simulink model "CMU_BORG_AplysiaModularNeuromechanics"  (R2024a)
settings: Solver=ode23  StartTime=0.0  StopTime=tend  FixedStep=0.001  MaxStep=0.1  RelTol=0.00001  AbsTol=0.0001
values from neighbouring files (symbols this model uses):
  B20_0 = 0    [ParameterRecalculation.m]    (also in ReferenceGeometry_and_Initialization.m)
  B31B32_0 = 0    [GetSteadyState.m]    (also in ParameterRecalculation.m = 1; ReferenceGeometry_and_Initialization.m = 1; VaryingSeaweedStrength.m = 1)
  B38_0 = 0    [ParameterRecalculation.m]    (also in ReferenceGeometry_and_Initialization.m)
  B40B30_0 = 0    [ParameterRecalculation.m]    (also in ReferenceGeometry_and_Initialization.m)
  B40B30_offTime_0 = 0    [ParameterRecalculation.m]    (also in ReferenceGeometry_and_Initialization.m)
  B43B45_0 = 0    [ParameterRecalculation.m]    (also in ReferenceGeometry_and_Initialization.m)
  B4B5_0 = 0    [ParameterRecalculation.m]    (also in ReferenceGeometry_and_Initialization.m)
  B64_0 = 1    [GetSteadyState.m]    (also in ParameterRecalculation.m = 0; ReferenceGeometry_and_Initialization.m = 0; VaryingSeaweedStrength.m = 0)
  B6B9B3_0 = 1    [GetSteadyState.m]    (also in ParameterRecalculation.m = 0; ReferenceGeometry_and_Initialization.m = 0; VaryingSeaweedStrength.m = 0)
  B7_0 = 0    [ParameterRecalculation.m]    (also in ReferenceGeometry_and_Initialization.m)
  B8_0 = 0    [ParameterRecalculation.m]    (also in ReferenceGeometry_and_Initialization.m)
  C1_0 = 0    [ParameterRecalculation.m]    (also in ReferenceGeometry_and_Initialization.m)
  C2_0 = 0    [ParameterRecalculation.m]    (also in ReferenceGeometry_and_Initialization.m)
  C6_0 = 0    [ParameterRecalculation.m]    (also in ReferenceGeometry_and_Initialization.m)
  C_theta = C_xg/(2*pi)    [ParameterRecalculation.m]    (also in ReferenceGeometry_and_Initialization.m = 0.000813600069086)
  C_xd = C_xg    [ParameterRecalculation.m]    (also in ReferenceGeometry_and_Initialization.m = 0.005112)
  C_xg = (1/inv_C(kk))*time_scaler*force_scaler    [DampingParameterConvergence.m]    (also in ReferenceGeometry_and_Initialization.m = 0.005112)
  C_xv = C_xd    [ParameterRecalculation.m]    (also in ReferenceGeometry_and_Initialization.m = 0.005112)
  C_yg = C_xg    [ParameterRecalculation.m]    (also in ReferenceGeometry_and_Initialization.m = 0.005112)
  CBI2_0 = 0    [ParameterRecalculation.m]    (also in ReferenceGeometry_and_Initialization.m)
  CBI3_0 = 0    [GetSteadyState.m]    (also in ParameterRecalculation.m = 1; ReferenceGeometry_and_Initialization.m = 1; VaryingSeaweedStrength.m = 1)
  CBI3_refractory_0 = 0    [ParameterRecalculation.m]    (also in ReferenceGeometry_and_Initialization.m)
  CBI3_stimOFF_0 = 0    [ParameterRecalculation.m]    (also in ReferenceGeometry_and_Initialization.m)
  CBI3_stimON_0 = 0    [ParameterRecalculation.m]    (also in ReferenceGeometry_and_Initialization.m)
  CBI4_0 = 0    [ParameterRecalculation.m]    (also in ReferenceGeometry_and_Initialization.m)
  E1_params = [AE10,TE10,tau_E1,L0_E1,Lmax_E1]    [ParameterRecalculation.m]    (also in ReferenceGeometry_and_Initialization.m)
  E2_params = [AE20,TE20,tau_E2,L0_E2,Lmax_E2]    [ParameterRecalculation.m]    (also in ReferenceGeometry_and_Initialization.m)
  E6_params = [AE60,TE60,tau_E6,L0_E6,Lmax_E6]    [ParameterRecalculation.m]    (also in ReferenceGeometry_and_Initialization.m)
  FE1_max = force_scaler*0.2    [ParameterRecalculation.m]    (also in ReferenceGeometry_and_Initialization.m = 0.048)
  FE2_max = FE1_max    [ParameterRecalculation.m]    (also in ReferenceGeometry_and_Initialization.m = 0.048)
  FE6_max = FE1_max    [ParameterRecalculation.m]    (also in ReferenceGeometry_and_Initialization.m = 0.048)
  FHinge_max = force_scaler*0.292    [ParameterRecalculation.m]    (also in ReferenceGeometry_and_Initialization.m = 0.07008)
  FI1d_max = force_scaler*3.2    [ParameterRecalculation.m]    (also in ReferenceGeometry_and_Initialization.m = 0.768)
  FI1v_max = FI1d_max    [ParameterRecalculation.m]    (also in ReferenceGeometry_and_Initialization.m = 0.768)
  FI2_max = force_scaler*1    [ParameterRecalculation.m]    (also in ReferenceGeometry_and_Initialization.m = 0.24)
  FI3_ant_max = force_scaler*0.1    [ParameterRecalculation.m]    (also in ReferenceGeometry_and_Initialization.m = 0.024)
  FI3_max = force_scaler*3    [ParameterRecalculation.m]    (also in ReferenceGeometry_and_Initialization.m = 0.72)
  FI4_max = force_scaler*0.9    [ParameterRecalculation.m]    (also in ReferenceGeometry_and_Initialization.m = 0.216)
  fixation_type = 0    [GetSteadyState.m]    (also in ModelController.m; VaryingSeaweedStrength.m)
  grasperR = 1    [ReferenceGeometry_and_Initialization.m]
  H_lumen = mean([L_jaw,L_LG]) / R_ref    [ReferenceGeometry_and_Initialization.m]
  Hinge_params = [A_hinge0,T_hinge0,tau_hinge,L0_hinge,Lmax_hinge]    [ParameterRecalculation.m]    (also in ReferenceGeometry_and_Initialization.m)
  I1d_params = [AI1d0,TI1d0,tau_I1d,L0_I1d,Lmax_I1d]    [ParameterRecalculation.m]    (also in ReferenceGeometry_and_Initialization.m)
  I1v_params = [AI1v0,TI1v0,tau_I1v,L0_I1v,Lmax_I1v]    [ParameterRecalculation.m]    (also in ReferenceGeometry_and_Initialization.m)
  I2_params = [AI20,TI20,tau_I2_ingestive,tau_I2_egestive,L0_I2,Lmax_I2]    [ParameterRecalculation.m]    (also in ReferenceGeometry_and_Initialization.m)
  I3_params = [AI30,TI30,tau_I3]    [ParameterRecalculation.m]    (also in ReferenceGeometry_and_Initialization.m)
  I3ant_params = [AI3_ant0,TI3_ant0,tau_I3ant]    [ParameterRecalculation.m]    (also in ReferenceGeometry_and_Initialization.m)
  I4_params = [AI40,TI40,tau_I4]    [ParameterRecalculation.m]    (also in ReferenceGeometry_and_Initialization.m)
  K_const = force_scaler*0.5    [ParameterRecalculation.m]    (also in ReferenceGeometry_and_Initialization.m = 0.12)
  K_Eso = force_scaler*0.01    [ParameterRecalculation.m]    (also in ReferenceGeometry_and_Initialization.m = 0.0024)
  K_H = force_scaler*2    [ParameterRecalculation.m]    (also in ReferenceGeometry_and_Initialization.m = 0.48)
  L0_eso = abs(xd0)    [ReferenceGeometry_and_Initialization.m]
  L0_H = 0    [ReferenceGeometry_and_Initialization.m]
  L0_I1d = L1d0    [ParameterRecalculation.m]    (also in ReferenceGeometry_and_Initialization.m)
  L0_I1v = L1v0    [ParameterRecalculation.m]    (also in ReferenceGeometry_and_Initialization.m)
  L_head = 0.82*tracing_scale_factor    [ReferenceGeometry_and_Initialization.m]
  MCC_0 = 1    [DampingParameterConvergence.m]    (also in ModelController.m; ParameterRecalculation.m = 0; ReferenceGeometry_and_Initialization.m = 0)
  params = param_vec    [ParameterRecalculation.m]    (also in ReferenceGeometry_and_Initialization.m)
  seaweed_strength = 1e6    (= 1000000)    [ModelController.m]    (also in VaryingSeaweedStrength.m = seaweed_strength_vec(ind))
  sens_chemical_lips = 0    [GetSteadyState.m]    (also in ModelController.m = 1; VaryingSeaweedStrength.m = 1)
  sens_mechanical_grasper = 1    [GetSteadyState.m]    (also in ModelController.m = 0; VaryingSeaweedStrength.m)
  sens_mechanical_lips = 1    [GetSteadyState.m]    (also in ModelController.m; VaryingSeaweedStrength.m)
  t_switch_chem_lips = 1e6    (= 1000000)    [GetSteadyState.m]    (also in ModelController.m = 54; VaryingSeaweedStrength.m)
  t_switch_fixation = 1e6    (= 1000000)    [GetSteadyState.m]    (also in ModelController.m = 30; VaryingSeaweedStrength.m = 4)
  t_switch_mech_grasp = 1e6    (= 1000000)    [GetSteadyState.m]    (also in ModelController.m = 10; VaryingSeaweedStrength.m)
  t_switch_mech_lips = 1e6    (= 1000000)    [GetSteadyState.m]    (also in ModelController.m; VaryingSeaweedStrength.m)
  theta_fg = buccal_mass_data(7)    [PlotModel.m]    (also in ReferenceGeometry_and_Initialization.m = -(head_outline{4,"Angle"} - head_outline{3,"Angle"})*(pi/180)
  theta_g0 = (180-(head_outline{3,"Angle"} + rot_global +5))*(pi/180)    [ReferenceGeometry_and_Initialization.m]
  theta_H = buccal_mass_data(6)    [PlotModel.m]    (also in ReferenceGeometry_and_Initialization.m = pi + theta_H_tilde - theta_g0)
  time_scaler = 1    [DampingParameterConvergence.m]    (also in ReferenceGeometry_and_Initialization.m = 1.065)
  ukg = 0.95*usg    (= 0.95)    [ParameterRecalculation.m]    (also in ReferenceGeometry_and_Initialization.m)
  ukh = 0.75*ush    (= 0.75)    [ParameterRecalculation.m]    (also in ReferenceGeometry_and_Initialization.m)
  usg = 1    [ParameterRecalculation.m]    (also in ReferenceGeometry_and_Initialization.m)
  ush = 1    [ParameterRecalculation.m]    (also in ReferenceGeometry_and_Initialization.m)
  xd0 = L_head - L1d0    [ReferenceGeometry_and_Initialization.m]
  xg0 = L_head + L_CG * cosd(a_CG) + 0.3    [ReferenceGeometry_and_Initialization.m]
  xh0 = 0    [ReferenceGeometry_and_Initialization.m]
  xv0 = L_head - L1v0    [ReferenceGeometry_and_Initialization.m]
  yg0 = L_CG * sind(a_CG) + 0.4    [ReferenceGeometry_and_Initialization.m]
(part 2 of 4)

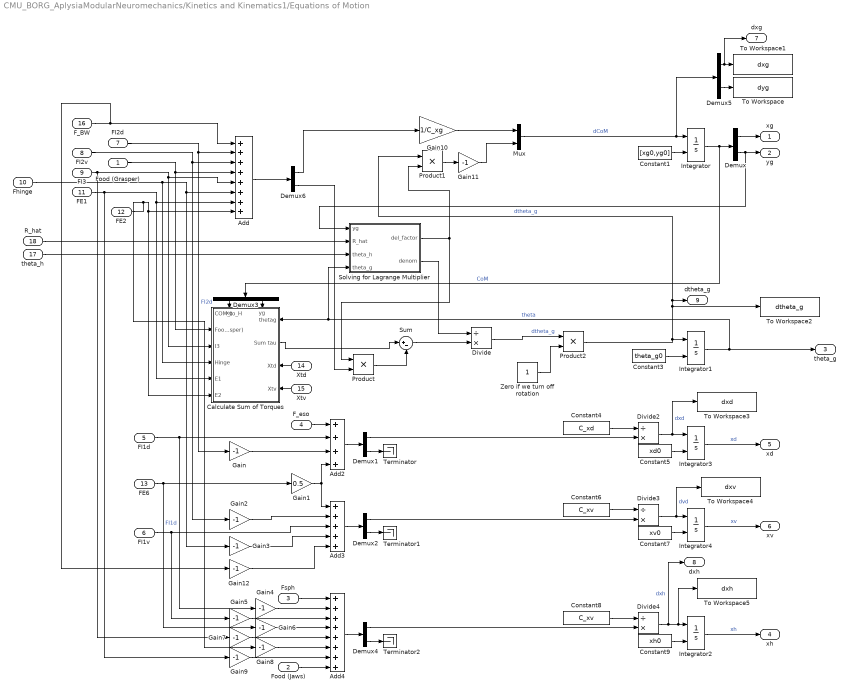
== system CMU_BORG_AplysiaModularNeuromechanics/Kinetics and Kinematics1/Equations of Motion ==
  Food (Grasper) : Inport
  Food (Jaws) : Inport  Port=2
  Fsph : Inport  Port=3
  F_eso : Inport  Port=4
  FI1d : Inport  Port=5
  FI1v : Inport  Port=6
  FI2d : Inport  Port=7
  FI2v : Inport  Port=8
  FI3 : Inport  Port=9
  Fhinge : Inport  Port=10
  FE1 : Inport  Port=11
  FE2 : Inport  Port=12
  FE6 : Inport  Port=13
  Xtd : Inport  Port=14
  Xtv : Inport  Port=15
  F_BW : Inport  Port=16
  theta_h : Inport  Port=17
  R_hat : Inport  Port=18
  Add : Sum  Inputs=++++++++
  Add2 : Sum  Inputs=++++
  Add3 : Sum  Inputs=+++++
  Add4 : Sum  Inputs=++++++++
  Calculate Sum of Torques : Subsystem
      settings: PortSchema="{\"entries\":[{\"content\":{\"sides\":[{\"content\":{\"connectorIds\":[\"Out2\",\"In1\",\"In2\",\"In3\",\"In4\",\"In5\"]},\"type\":\"ConnectorPlacement.EquallySpacedRectSide\",\"uuid\":\"c0e43481-c216-4ad4-881f-d2fdf68e5ec3\"},{\"content\":{\"connectorIds\":[\"In8\",\"Out1\",\"In9\",\"In10\"],\"side\":\"RIGHT\"},\"type\":\"ConnectorPlacement.EquallySpacedRectSide\",\"uuid\":\"16d7448a-0f3e-4f3f-aeff-70fb4c79f422\"},{\"content\":{\"connectorIds\":[\"In6\",\"In7\"],\"side\":\"TOP\"},\"type\":\"ConnectorPlacement.EquallySpacedRectSide\",\"uuid\":\"c05223d0-8379-44e5-9257-55939348b923\"},{\"content\":{\"connectorIds\":[],\"side\":\"BOTTOM\"},\"type\":\"ConnectorPlacement.EquallySpacedRectSide\",\"uuid\":\"e93484de-b6f0-4451-adeb-54f3491074ac\"}]},\"type\":\"ConnectorPlacement.EquallySpacedConnector\",\"uuid\":\"67ed4a1a-6673-493c-bdea-c21b4d7fd3f4\"}],\"packageUris\":[\"http://schema.mathworks.com/mf0/Connector/R2020b\"],\"version\":\"1.0\"}"
  Constant1 : Constant  Value=[xg0,yg0]
  Constant3 : Constant  Value=theta_g0
  Constant4 : Constant  Value=C_xd
  Constant5 : Constant  Value=xd0
  Constant6 : Constant  Value=C_xv
  Constant7 : Constant  Value=xv0
  Constant8 : Constant  Value=C_xv
  Constant9 : Constant  Value=xh0
  Demux{,1..6} (7 alike) : Demux  Outputs=2
  Divide{,2..4} (4 alike) : Product  Inputs=/*
  Gain{,2..9,11..12} (11 alike) : Gain  Gain=-1
  Gain1 : Gain  Gain=0.5
  Gain10 : Gain  Gain=1/C_xg
  Integrator{,1..4} (5 alike) : Integrator  InitialConditionSource=external
  Mux : Mux  Inputs=2
  Product : Product
  Product1 : Product
  Product2 : Product
  Solving for Lagrange Multiplier : Subsystem
  Sum : Sum  Inputs=|+-
  Terminator : Terminator
  Terminator1 : Terminator
  Terminator2 : Terminator
  To Workspace : ToWorkspace  VariableName=dyg  SampleTime=-1
  To Workspace1 : ToWorkspace  VariableName=dxg  SampleTime=-1
  To Workspace2 : ToWorkspace  VariableName=dtheta_g  SampleTime=-1
  To Workspace3 : ToWorkspace  VariableName=dxd  SampleTime=-1
  To Workspace4 : ToWorkspace  VariableName=dxv  SampleTime=-1
  To Workspace5 : ToWorkspace  VariableName=dxh  SampleTime=-1
  Zero if we turn off rotation : Constant  OutDataTypeStr=Inherit: Inherit via back propagation
  xg : Outport
  yg : Outport  Port=2
  theta_g : Outport  Port=3
  xh : Outport  Port=4
  xd : Outport  Port=5
  xv : Outport  Port=6
  dxg : Outport  Port=7
  dxh : Outport  Port=8
  dtheta_g : Outport  Port=9
  wires:
  Integrator/1 -> Demux3/1, Demux/1  "CoM"
  Demux/1 -> xg/1
  Demux/2 -> Solving for Lagrange Multiplier/1(yg), yg/1
  Integrator1/1 -> Solving for Lagrange Multiplier/4(theta_g), Calculate Sum of Torques/8(thetag), theta_g/1  "theta"
  Integrator2/1 -> xh/1  "xh"
  Integrator3/1 -> xd/1  "xd"
  Integrator4/1 -> xv/1  "xv"
  Mux/1 -> Demux5/1, Integrator/1  "dCoM"
  Constant1/1 -> Integrator/2
  FI2d/1 -> Add/2, Gain/1  "FI2d"
  FI2v/1 -> Add/3, Gain2/1
  Food (Grasper)/1 -> Add/4, Calculate Sum of Torques/1(Food (Grasper))
  FI3/1 -> Gain7/1, Add/5, Calculate Sum of Torques/2(I3)
  Fhinge/1 -> Calculate Sum of Torques/3(Hinge), Add/6, Gain3/1
  FE1/1 -> Gain9/1, Add/7, Calculate Sum of Torques/4(E1)
  FE2/1 -> Gain8/1, Add/8, Calculate Sum of Torques/5(E2)
  Constant3/1 -> Integrator1/2
  Constant4/1 -> Divide2/1
  Divide2/1 -> To Workspace3/1, Integrator3/1  "dxd"
  Constant5/1 -> Integrator3/2
  Constant6/1 -> Divide3/1
  Constant7/1 -> Integrator4/2
  Divide3/1 -> To Workspace4/1, Integrator4/1  "dvd"
  Add2/1 -> Demux1/1
  Demux1/2 -> Terminator/1
  Demux1/1 -> Divide2/2
  Demux2/2 -> Terminator1/1
  Add3/1 -> Demux2/1
  Demux2/1 -> Divide3/2
  F_eso/1 -> Add2/1
  FI1d/1 -> Gain4/1, Add2/2  "FI1d"
  Gain/1 -> Add2/3
  FE6/1 -> Gain6/1, Gain1/1
  Gain1/1 -> Add3/1, Add2/4
  FI1v/1 -> Gain5/1, Add3/3
  Gain3/1 -> Add3/4
  Gain2/1 -> Add3/2
  Demux3/1 -> Calculate Sum of Torques/6(xg)
  Demux3/2 -> Calculate Sum of Torques/7(yg)
  Xtd/1 -> Calculate Sum of Torques/9(Xtd)
  Xtv/1 -> Calculate Sum of Torques/10(Xtv)
  Demux4/1 -> Divide4/2
  Divide4/1 -> dxh/1, To Workspace5/1, Integrator2/1  "dxh"
  Constant8/1 -> Divide4/1
  Constant9/1 -> Integrator2/2
  Demux4/2 -> Terminator2/1
  Add4/1 -> Demux4/1
  Fsph/1 -> Add4/1
  Gain4/1 -> Add4/2
  Gain5/1 -> Add4/3
  Gain6/1 -> Add4/4
  Gain7/1 -> Add4/5
  Gain8/1 -> Add4/6
  Food (Jaws)/1 -> Add4/8
  Gain9/1 -> Add4/7
  Demux5/1 -> dxg/1, To Workspace1/1
  Demux5/2 -> To Workspace/1
  Add/1 -> Demux6/1
  Demux6/1 -> Gain10/1
  Product1/1 -> Gain11/1
  Gain10/1 -> Mux/1
  Calculate Sum of Torques/1(Sum tau) -> Sum/1
  Product/1 -> Sum/2
  Demux6/2 -> Product/2
  Solving for Lagrange Multiplier/1(del_factor) -> Product1/2, Product/1
  Sum/1 -> Divide/2
  Solving for Lagrange Multiplier/2(denom) -> Divide/1
  Product2/1 -> dtheta_g/1, Product1/1, To Workspace2/1, Integrator1/1  "dtheta_g"
  Gain11/1 -> Mux/2
  Divide/1 -> Product2/1  "dtheta_g"
  Zero if we turn off rotation/1 -> Product2/2
  R_hat/1 -> Solving for Lagrange Multiplier/2(R_hat)
  theta_h/1 -> Solving for Lagrange Multiplier/3(theta_h)
  F_BW/1 -> Add/1, Gain12/1
  Gain12/1 -> Add3/5

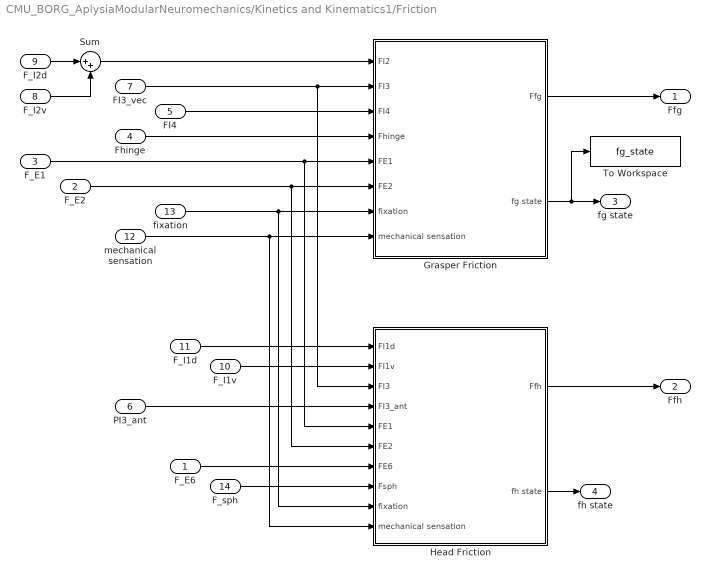
== system CMU_BORG_AplysiaModularNeuromechanics/Kinetics and Kinematics1/Friction ==
  F_E6 : Inport
  F_E2 : Inport  Port=2
  F_E1 : Inport  Port=3
  Fhinge : Inport  Port=4
  FI4 : Inport  Port=5
  PI3_ant : Inport  Port=6
  FI3_vec : Inport  Port=7
  F_I2v : Inport  Port=8
  F_I2d : Inport  Port=9
  F_I1v : Inport  Port=10
  F_I1d : Inport  Port=11
  mechanical sensation : Inport  Port=12
  fixation : Inport  Port=13
  F_sph : Inport  Port=14
  Grasper Friction : Subsystem
  Head Friction : Subsystem
  Sum : Sum  Inputs=|++
  To Workspace : ToWorkspace  VariableName=fg_state  SampleTime=-1
  Ffg : Outport
  Ffh : Outport  Port=2
  fg state : Outport  Port=3
  fh state : Outport  Port=4
  wires:
  PI3_ant/1 -> Head Friction/4(FI3_ant)
  mechanical sensation/1 -> Head Friction/10(mechanical sensation), Grasper Friction/8(mechanical sensation)
  fixation/1 -> Head Friction/9(fixation), Grasper Friction/7(fixation)
  Fhinge/1 -> Grasper Friction/4(Fhinge)
  FI4/1 -> Grasper Friction/3(FI4)
  FI3_vec/1 -> Head Friction/3(FI3), Grasper Friction/2(FI3)
  Sum/1 -> Grasper Friction/1(FI2)
  Head Friction/2(fh state) -> fh state/1
  Grasper Friction/2(fg state) -> To Workspace/1, fg state/1
  Grasper Friction/1(Ffg) -> Ffg/1
  Head Friction/1(Ffh) -> Ffh/1
  F_I2d/1 -> Sum/1
  F_I2v/1 -> Sum/2
  F_E1/1 -> Head Friction/5(FE1), Grasper Friction/5(FE1)
  F_E2/1 -> Head Friction/6(FE2), Grasper Friction/6(FE2)
  F_I1v/1 -> Head Friction/2(FI1v)
  F_I1d/1 -> Head Friction/1(FI1d)
  F_E6/1 -> Head Friction/7(FE6)
  F_sph/1 -> Head Friction/8(Fsph)

== system CMU_BORG_AplysiaModularNeuromechanics/Kinetics and Kinematics1/I3 Body Wall Contact Force ==
  xv : Inport
  yg : Inport  Port=2
  xg : Inport  Port=3
  x_hinge : Inport  Port=4
  Constant : Constant  Value=grasperR
  MATLAB Function : MATLAB Function  TreatAsAtomicUnit=on
  F_BW : Outport
  wires:
  xv/1 -> MATLAB Function/4(xv)
  xg/1 -> MATLAB Function/1(xg)
  yg/1 -> MATLAB Function/2(yg)
  x_hinge/1 -> MATLAB Function/3(x_hinge)
  MATLAB Function/1(F) -> F_BW/1
  Constant/1 -> MATLAB Function/5(R)

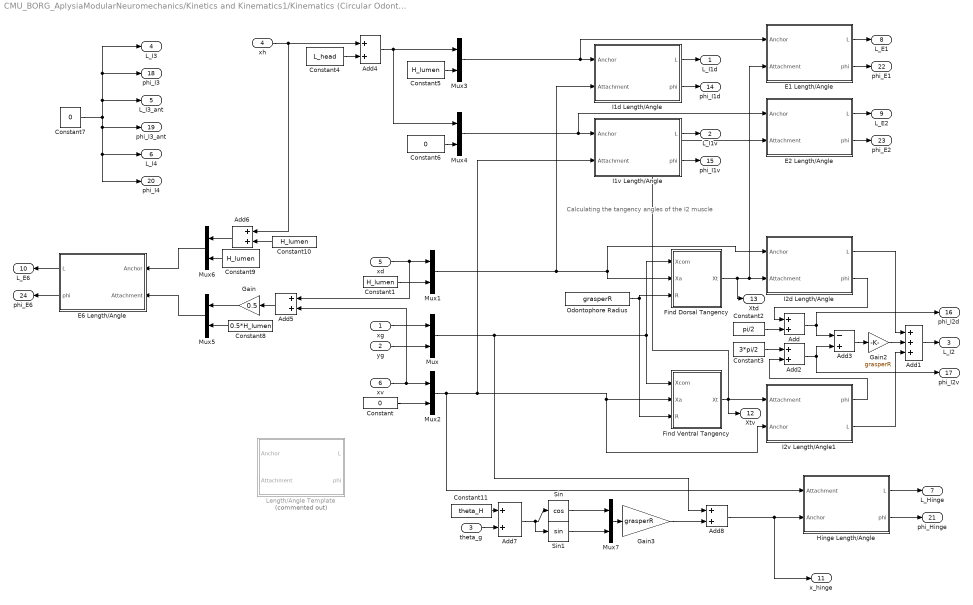
== system CMU_BORG_AplysiaModularNeuromechanics/Kinetics and Kinematics1/Kinematics (Circular Odontophore) ==
  note: Calculating the tangency angles of the I2 muscle
  xg : Inport
  yg : Inport  Port=2
  theta_g : Inport  Port=3
  xh : Inport  Port=4
  xd : Inport  Port=5
  xv : Inport  Port=6
  Add{,2,4..8} (7 alike) : Sum
  Add1 : Sum  Inputs=+++
  Add3 : Sum  Inputs=-+
  Constant : Constant  Value=0
  Constant{1,5,9..10} (4 alike) : Constant  Value=H_lumen
  Constant11 : Constant  Value=theta_H
  Constant2 : Constant  Value=pi/2
  Constant3 : Constant  Value=3*pi/2
  Constant4 : Constant  Value=L_head
  Constant6 : Constant  Value=0
  Constant7 : Constant  Value=0
  Constant8 : Constant  Value=0.5*H_lumen
  E1 Length/Angle : Subsystem
  E2 Length/Angle : Subsystem
  E6 Length/Angle : Subsystem
  Find Dorsal Tangency : MATLAB Function  TreatAsAtomicUnit=on
  Find Ventral Tangency : MATLAB Function  TreatAsAtomicUnit=on
  Gain : Gain  Gain=0.5
  Gain2 : Gain  Gain=grasperR
  Gain3 : Gain  Gain=grasperR
  Hinge Length/Angle : Subsystem
  I1d Length/Angle : Subsystem
  I1v Length/Angle : Subsystem
  I2d Length/Angle : Subsystem
  I2v Length/Angle1 : Subsystem
  Length/Angle Template : Subsystem  Commented=on
  Mux{,1..7} (8 alike) : Mux  Inputs=2
  Odontophore Radius : Constant  Value=grasperR
  Sin : Trigonometry  Operator=cos
  Sin1 : Trigonometry
  L_I1d : Outport
  L_I1v : Outport  Port=2
  L_I2 : Outport  Port=3
  L_I3 : Outport  Port=4
  L_I3_ant : Outport  Port=5
  L_I4 : Outport  Port=6
  L_Hinge : Outport  Port=7
  L_E1 : Outport  Port=8
  L_E2 : Outport  Port=9
  L_E6 : Outport  Port=10
  x_hinge : Outport  Port=11
  Xtv : Outport  Port=12
  Xtd : Outport  Port=13
  phi_I1d : Outport  Port=14
  phi_I1v : Outport  Port=15
  phi_I2d : Outport  Port=16
  phi_I2v : Outport  Port=17
  phi_I3 : Outport  Port=18
  phi_I3_ant : Outport  Port=19
  phi_I4 : Outport  Port=20
  phi_Hinge : Outport  Port=21
  phi_E1 : Outport  Port=22
  phi_E2 : Outport  Port=23
  phi_E6 : Outport  Port=24
  wires:
  Gain2/1 -> Add1/2
  Add3/1 -> Gain2/1
  Odontophore Radius/1 -> Find Ventral Tangency/3(R), Find Dorsal Tangency/3(R)
  xg/1 -> Mux/1
  yg/1 -> Mux/2
  xd/1 -> Add5/1, Mux1/1
  xv/1 -> Add5/2, Mux2/1
  Constant/1 -> Mux2/2
  Constant1/1 -> Mux1/2
  Mux/1 -> Find Ventral Tangency/1(Xcom), Find Dorsal Tangency/1(Xcom), Add8/1
  Mux1/1 -> I1d Length/Angle/2(Attachment), Find Dorsal Tangency/2(Xa), I2d Length/Angle/1(Anchor)
  Mux2/1 -> I2v Length/Angle1/2(Anchor), Find Ventral Tangency/2(Xa), I1v Length/Angle/2(Attachment), Hinge Length/Angle/1(Attachment)
  Find Dorsal Tangency/1(Xt) -> Xtd/1, I2d Length/Angle/2(Attachment), E1 Length/Angle/2(Attachment)
  Find Ventral Tangency/1(Xt) -> Xtv/1, I2v Length/Angle1/1(Attachment), E2 Length/Angle/2(Attachment)
  I2d Length/Angle/1(L) -> Add1/1
  I2v Length/Angle1/2(L) -> Add1/3
  Add1/1 -> L_I2/1
  I2d Length/Angle/2(phi) -> Add/1
  Constant2/1 -> Add/2
  I2v Length/Angle1/1(phi) -> Add2/2
  Constant3/1 -> Add2/1
  Add2/1 -> phi_I2v/1, Add3/2
  Add/1 -> phi_I2d/1, Add3/1
  xh/1 -> Add6/1, Add4/1
  Constant4/1 -> Add4/2
  Constant5/1 -> Mux3/2
  Mux3/1 -> E1 Length/Angle/1(Anchor), I1d Length/Angle/1(Anchor)
  Mux4/1 -> E2 Length/Angle/1(Anchor), I1v Length/Angle/1(Anchor)
  Constant6/1 -> Mux4/2
  Add4/1 -> Mux4/1, Mux3/1
  I1d Length/Angle/1(L) -> L_I1d/1
  I1v Length/Angle/1(L) -> L_I1v/1
  I1d Length/Angle/2(phi) -> phi_I1d/1
  I1v Length/Angle/2(phi) -> phi_I1v/1
  E1 Length/Angle/2(phi) -> phi_E1/1
  E1 Length/Angle/1(L) -> L_E1/1
  E2 Length/Angle/1(L) -> L_E2/1
  E2 Length/Angle/2(phi) -> phi_E2/1
  Constant7/1 -> phi_I3_ant/1, L_I4/1, phi_I4/1, L_I3_ant/1, phi_I3/1, L_I3/1
  Add5/1 -> Gain/1
  Gain/1 -> Mux5/1
  Constant8/1 -> Mux5/2
  Mux5/1 -> E6 Length/Angle/2(Attachment)
  Constant9/1 -> Mux6/2
  Add6/1 -> Mux6/1
  Constant10/1 -> Add6/2
  Mux6/1 -> E6 Length/Angle/1(Anchor)
  E6 Length/Angle/1(L) -> L_E6/1
  E6 Length/Angle/2(phi) -> phi_E6/1
  theta_g/1 -> Add7/2
  Constant11/1 -> Add7/1
  Sin/1 -> Mux7/1
  Add7/1 -> Sin1/1, Sin/1
  Mux7/1 -> Gain3/1
  Gain3/1 -> Add8/2
  Add8/1 -> x_hinge/1, Hinge Length/Angle/2(Anchor)
  Hinge Length/Angle/1(L) -> L_Hinge/1
  Hinge Length/Angle/2(phi) -> phi_Hinge/1
  Sin1/1 -> Mux7/2

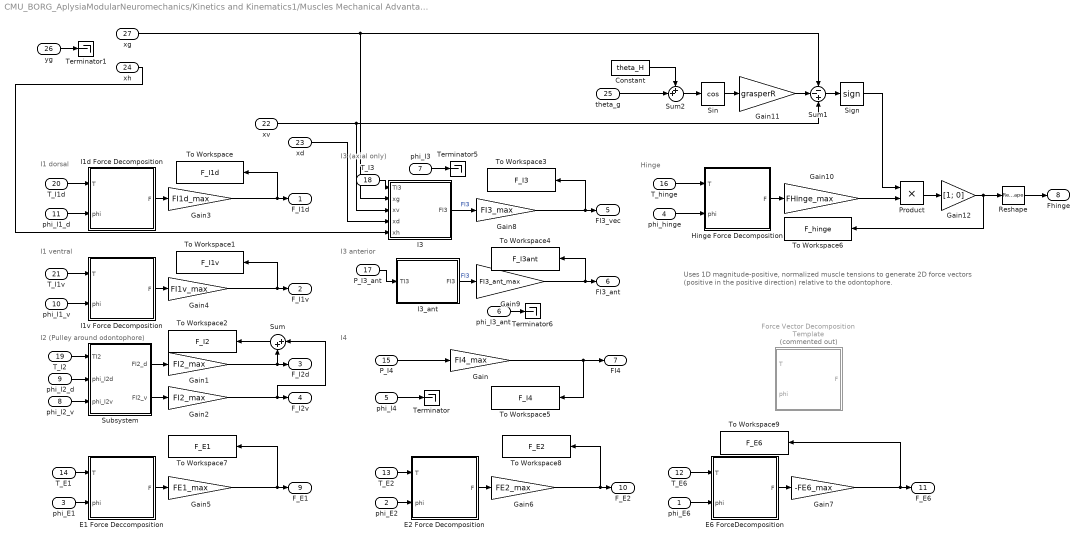
== system CMU_BORG_AplysiaModularNeuromechanics/Kinetics and Kinematics1/Muscles Mechanical Advantage Module ==
  note: I1 dorsal
  note: I1 ventral
  note: Uses 1D magnitude-positive, normalized muscle tensions to generate 2D force vectors (positive in the positive direction) relative to the odontophore.
  note: I3 (axial only)
  note: Hinge
  note: I2 (Pulley around odontophore)
  note: I4
  note: I3 anterior
  phi_E6 : Inport
  phi_E2 : Inport  Port=2
  phi_E1 : Inport  Port=3
  phi_hinge : Inport  Port=4
  phi_I4 : Inport  Port=5
  phi_I3_ant : Inport  Port=6
  phi_I3 : Inport  Port=7
  phi_I2_v : Inport  Port=8
  phi_I2_d : Inport  Port=9
  phi_I1_v : Inport  Port=10
  phi_I1_d : Inport  Port=11
  T_E6 : Inport  Port=12
  T_E2 : Inport  Port=13
  T_E1 : Inport  Port=14
  P_I4 : Inport  Port=15
  T_hinge : Inport  Port=16
  P_I3_ant : Inport  Port=17
  T_I3 : Inport  Port=18
  T_I2 : Inport  Port=19
  T_I1d : Inport  Port=20
  T_I1v : Inport  Port=21
  xv : Inport  Port=22
  xd : Inport  Port=23
  xh : Inport  Port=24
  theta_g : Inport  Port=25
  yg : Inport  Port=26
  xg : Inport  Port=27
  Constant : Constant  Value=theta_H
  E1 Force Deccomposition : Subsystem
  E2 Force Decomposition : Subsystem
  E6 ForceDecomposition : Subsystem
  Force Vector Decomposition Template : Subsystem  Commented=on
  Gain : Gain  Gain=FI4_max
  Gain1 : Gain  Gain=FI2_max
  Gain10 : Gain  Gain=FHinge_max
  Gain11 : Gain  Gain=grasperR
  Gain12 : Gain  Gain=[1; 0]
  Gain2 : Gain  Gain=FI2_max
  Gain3 : Gain  Gain=FI1d_max
  Gain4 : Gain  Gain=FI1v_max
  Gain5 : Gain  Gain=FE1_max
  Gain6 : Gain  Gain=FE2_max
  Gain7 : Gain  Gain=-FE6_max
  Gain8 : Gain  Gain=FI3_max
  Gain9 : Gain  Gain=FI3_ant_max
  Hinge Force Decomposition : Subsystem
  I1d Force Decomposition : Subsystem
  I1v Force Decomposition : Subsystem
  I3 : Subsystem
  I3_ant : Subsystem
  Product : Product
  Reshape : Reshape  OutputDimensionality=Customize  OutputDimensions=2
  Sign : Signum
  Sin : Trigonometry  Operator=cos
  Subsystem : Subsystem
  Sum : Sum  Inputs=|++
  Sum1 : Sum  Inputs=--+
  Sum2 : Sum  Inputs=++|
  Terminator{,1,5..6} (4 alike) : Terminator
  To Workspace : ToWorkspace  VariableName=F_I1d  SampleTime=-1
  To Workspace1 : ToWorkspace  VariableName=F_I1v  SampleTime=-1
  To Workspace2 : ToWorkspace  VariableName=F_I2  SampleTime=-1
  To Workspace3 : ToWorkspace  VariableName=F_I3  SampleTime=-1
  To Workspace4 : ToWorkspace  VariableName=F_I3ant  SampleTime=-1
  To Workspace5 : ToWorkspace  VariableName=F_I4  SampleTime=-1
  To Workspace6 : ToWorkspace  VariableName=F_hinge  SampleTime=-1
  To Workspace7 : ToWorkspace  VariableName=F_E1  SampleTime=-1
  To Workspace8 : ToWorkspace  VariableName=F_E2  SampleTime=-1
  To Workspace9 : ToWorkspace  VariableName=F_E6  SampleTime=-1
  F_I1d : Outport
  F_I1v : Outport  Port=2
  F_I2d : Outport  Port=3
  F_I2v : Outport  Port=4
  FI3_vec : Outport  Port=5
  FI3_ant : Outport  Port=6
  FI4 : Outport  Port=7
  Fhinge : Outport  Port=8
  F_E1 : Outport  Port=9
  F_E2 : Outport  Port=10
  F_E6 : Outport  Port=11
  wires:
  Gain9/1 -> To Workspace4/1, FI3_ant/1
  Gain/1 -> To Workspace5/1, FI4/1
  P_I4/1 -> Gain/1
  Gain1/1 -> Sum/2, F_I2d/1
  phi_I2_v/1 -> Subsystem/3(phi_I2v)
  phi_I2_d/1 -> Subsystem/2(phi_I2d)
  Gain10/1 -> Product/2
  T_I2/1 -> Subsystem/1(TI2)
  T_I3/1 -> I3/1(TI3)
  Gain2/1 -> Sum/1, F_I2v/1
  Subsystem/1(FI2_d) -> Gain1/1
  Subsystem/2(FI2_v) -> Gain2/1
  T_I1v/1 -> I1v Force Decomposition/1(T)
  phi_I1_v/1 -> I1v Force Decomposition/2(phi)
  phi_I1_d/1 -> I1d Force Decomposition/2(phi)
  T_I1d/1 -> I1d Force Decomposition/1(T)
  I1d Force Decomposition/1(F) -> Gain3/1
  I1v Force Decomposition/1(F) -> Gain4/1
  Gain3/1 -> To Workspace/1, F_I1d/1
  Gain4/1 -> To Workspace1/1, F_I1v/1
  phi_E1/1 -> E1 Force Deccomposition/2(phi)
  T_E1/1 -> E1 Force Deccomposition/1(T)
  E1 Force Deccomposition/1(F) -> Gain5/1
  Gain5/1 -> To Workspace7/1, F_E1/1
  Gain6/1 -> To Workspace8/1, F_E2/1
  E2 Force Decomposition/1(F) -> Gain6/1
  T_E2/1 -> E2 Force Decomposition/1(T)
  phi_E2/1 -> E2 Force Decomposition/2(phi)
  phi_E6/1 -> E6 ForceDecomposition/2(phi)
  T_E6/1 -> E6 ForceDecomposition/1(T)
  E6 ForceDecomposition/1(F) -> Gain7/1
  Gain7/1 -> To Workspace9/1, F_E6/1
  phi_I4/1 -> Terminator/1
  yg/1 -> Terminator1/1
  xd/1 -> I3/4(xd)
  xv/1 -> Sum1/3, I3/3(xv)
  xg/1 -> Sum1/1, I3/2(xg)
  phi_I3/1 -> Terminator5/1
  Gain8/1 -> To Workspace3/1, FI3_vec/1
  I3/1(FI3) -> Gain8/1  "FI3"
  I3_ant/1(FI3) -> Gain9/1  "FI3"
  P_I3_ant/1 -> I3_ant/1(TI3)
  phi_I3_ant/1 -> Terminator6/1
  T_hinge/1 -> Hinge Force Decomposition/1(T)
  phi_hinge/1 -> Hinge Force Decomposition/2(phi)
  Hinge Force Decomposition/1(F) -> Gain10/1
  Sum/1 -> To Workspace2/1
  Sin/1 -> Gain11/1
  Gain11/1 -> Sum1/2
  Sum1/1 -> Sign/1
  Sum2/1 -> Sin/1
  theta_g/1 -> Sum2/2
  Constant/1 -> Sum2/1
  xh/1 -> I3/5(xh)
  Product/1 -> Gain12/1
  Gain12/1 -> To Workspace6/1, Reshape/1
  Sign/1 -> Product/1
  Reshape/1 -> Fhinge/1

== system CMU_BORG_AplysiaModularNeuromechanics/Kinetics and Kinematics1/Seaweed Breaking ==
  note: broken
  fixation : Inport
  F_food : Inport  Port=2
  Constant : Constant
  Constant1 : Constant  Value=seaweed_strength
  Constant2 : Constant  Value=0
  Constant3 : Constant  Value=0
  GreaterThan : RelationalOperator  Operator=>  OutDataTypeStr=boolean  RndMeth=Simplest  InputSameDT=off
  Memory : Memory
  OR : Logic  Operator=OR  IconShape=distinctive  AllPortsSameDT=off  OutDataTypeStr=boolean
  Switch : Switch  Criteria=u2 > Threshold  SaturateOnIntegerOverflow=off  InputSameDT=off
  Switch1 : Switch  Criteria=u2 > Threshold  SaturateOnIntegerOverflow=off  InputSameDT=off
  fixation_out : Outport
  wires:
  F_food/1 -> GreaterThan/1
  Constant1/1 -> GreaterThan/2
  GreaterThan/1 -> OR/1
  OR/1 -> Switch/2
  Switch/1 -> Switch1/2, Memory/1
  Constant/1 -> Switch/1
  Constant2/1 -> Switch/3
  fixation/1 -> Switch1/3
  Constant3/1 -> Switch1/1
  Switch1/1 -> fixation_out/1
  Memory/1 -> OR/2

== system CMU_BORG_AplysiaModularNeuromechanics/Kinetics and Kinematics1/Seaweed Ingestion Calculations ==
  note: True if the jaws are not preventing motion
  note: is there seaweed held in the grasper
  note: is I3_ant holding food in place
  note: is the grasper moving forward
  fg_state : Inport
  dxg : Inport  Port=2
  dthetag : Inport  Port=3
  thetag : Inport  Port=4
  FI3_ant : Inport  Port=5
  Constant : Constant  Value=grasperR
  Constant1 : Constant  Value=theta_fg
  Constant2 : Constant  Value=sens_mechanical_grasper
  Demux : Demux  Outputs=2
  Gain : Gain  Gain=-1
  Gain1 : Gain  Gain=1/FI3_ant_max
  Integrator : Integrator
  MATLAB Function : MATLAB Function  TreatAsAtomicUnit=on
  Scope : Scope
  Terminator : Terminator
  L_seaweed_ingested : Outport
  dxf : Outport  Port=2
  wires:
  Integrator/1 -> L_seaweed_ingested/1
  Gain/1 -> Integrator/1
  MATLAB Function/1(dL_ingested) -> Gain/1
  MATLAB Function/2(dxf) -> Scope/1, dxf/1
  thetag/1 -> MATLAB Function/3(thetag)
  Constant1/1 -> MATLAB Function/6(theta_fg)
  dthetag/1 -> MATLAB Function/2(dthetag)
  Constant/1 -> MATLAB Function/7(grasperR)
  dxg/1 -> MATLAB Function/1(dxg)
  fg_state/1 -> MATLAB Function/4(fg_state)
  Constant2/1 -> MATLAB Function/8(sense_mechanical_grasper)
  Gain1/1 -> MATLAB Function/5(FI3_ant_norm)
  Demux/1 -> Gain1/1
  FI3_ant/1 -> Demux/1
  Demux/2 -> Terminator/1

== system CMU_BORG_AplysiaModularNeuromechanics/Kinetics and Kinematics1/Springs ==
  xg : Inport
  yg : Inport  Port=2
  theta_g : Inport  Port=3
  xh : Inport  Port=4
  xd : Inport  Port=5
  xv : Inport  Port=6
  Esophagus Spring : Subsystem
  Grasper-Head Spring1 : Subsystem
  Terminator{,1..3} (4 alike) : Terminator
  F_eso : Outport
  Fsph : Outport  Port=2
  wires:
  Esophagus Spring/1(F_eso) -> F_eso/1  "F_eso"
  Grasper-Head Spring1/1(F_sph) -> Fsph/1
  xh/1 -> Grasper-Head Spring1/1(xh)
  xd/1 -> Esophagus Spring/1(xd)
  yg/1 -> Terminator/1
  theta_g/1 -> Terminator1/1
  xv/1 -> Terminator2/1
  xg/1 -> Terminator3/1

== system CMU_BORG_AplysiaModularNeuromechanics/Muscle Activation and Tension Module/E1 - First Order + Spring Muscle Model ==
  note: List of parameters:
      | 	- A_0: starting activation
      | 	- T_0: starting tension
      | 	- tau_i: intrinsic time constant of the muscle i
      | 	- L_0: rest length of muscle
      | 	- L_max: length of maximum force
  note: Passive Force
  note: Active Force Dynamics
  note: Neural Dynamics
  Motor Neuron In : Inport
  Muscle Length : Inport  Port=2
  Parameters : Inport  Port=3
  Add : Sum
  Demux : Demux  Outputs=5
  Divide : Product  Inputs=/*
  Divide1 : Product  Inputs=/*
  Divide2 : Product  Inputs=/*
  Integrator : Integrator  InitialConditionSource=external
  Integrator1 : Integrator  InitialConditionSource=external
  Subtract{,1..3} (4 alike) : Sum  Inputs=+-
  Switch : Switch  Criteria=u2 > Threshold  ZeroCross=off  SaturateOnIntegerOverflow=off  InputSameDT=off
  Zero : Constant  Value=0  OutDataTypeStr=Inherit: Inherit via back propagation
  Normalized Tension : Outport
  Activation : Outport  Port=2
  wires:
  Zero/1 -> Switch/3
  Switch/1 -> Add/2
  Divide2/1 -> Switch/1
  Muscle Length/1 -> Subtract3/1
  Parameters/1 -> Demux/1
  Motor Neuron In/1 -> Subtract/1
  Subtract/1 -> Divide/2
  Divide/1 -> Integrator/1
  Demux/3 -> Divide1/1, Divide/1
  Demux/1 -> Integrator/2
  Integrator/1 -> Subtract1/1, Subtract/2, Activation/1
  Subtract1/1 -> Divide1/2
  Divide1/1 -> Integrator1/1
  Demux/2 -> Integrator1/2
  Integrator1/1 -> Add/1, Subtract1/2
  Demux/5 -> Subtract2/1
  Demux/4 -> Subtract3/2, Subtract2/2
  Subtract2/1 -> Divide2/1
  Subtract3/1 -> Divide2/2, Switch/2
  Add/1 -> Normalized Tension/1

== system CMU_BORG_AplysiaModularNeuromechanics/Muscle Activation and Tension Module/E2 - First Order + Spring Muscle Model ==
  note: List of parameters:
      | 	- A_0: starting activation
      | 	- T_0: starting tension
      | 	- tau_i: intrinsic time constant of the muscle i
      | 	- L_0: rest length of muscle
      | 	- L_max: length of maximum force
  note: Passive Force
  note: Active Force Dynamics
  note: Neural Dynamics
  Motor Neuron In : Inport
  Muscle Length : Inport  Port=2
  Parameters : Inport  Port=3
  Add : Sum
  Demux : Demux  Outputs=5
  Divide : Product  Inputs=/*
  Divide1 : Product  Inputs=/*
  Divide2 : Product  Inputs=/*
  Integrator : Integrator  InitialConditionSource=external
  Integrator1 : Integrator  InitialConditionSource=external
  Subtract{,1..3} (4 alike) : Sum  Inputs=+-
  Switch : Switch  Criteria=u2 > Threshold  ZeroCross=off  SaturateOnIntegerOverflow=off  InputSameDT=off
  Zero : Constant  Value=0  OutDataTypeStr=Inherit: Inherit via back propagation
  Normalized Tension : Outport
  Activation : Outport  Port=2
  wires:
  Zero/1 -> Switch/3
  Switch/1 -> Add/2
  Divide2/1 -> Switch/1
  Muscle Length/1 -> Subtract3/1
  Parameters/1 -> Demux/1
  Motor Neuron In/1 -> Subtract/1
  Subtract/1 -> Divide/2
  Divide/1 -> Integrator/1
  Demux/3 -> Divide1/1, Divide/1
  Demux/1 -> Integrator/2
  Integrator/1 -> Subtract1/1, Subtract/2, Activation/1
  Subtract1/1 -> Divide1/2
  Divide1/1 -> Integrator1/1
  Demux/2 -> Integrator1/2
  Integrator1/1 -> Add/1, Subtract1/2
  Demux/5 -> Subtract2/1
  Demux/4 -> Subtract3/2, Subtract2/2
  Subtract2/1 -> Divide2/1
  Subtract3/1 -> Divide2/2, Switch/2
  Add/1 -> Normalized Tension/1

== system CMU_BORG_AplysiaModularNeuromechanics/Muscle Activation and Tension Module/E6 - First Order + Spring Muscle Model ==
  note: List of parameters:
      | 	- A_0: starting activation
      | 	- T_0: starting tension
      | 	- tau_i: intrinsic time constant of the muscle i
      | 	- L_0: rest length of muscle
      | 	- L_max: length of maximum force
  note: Passive Force
  note: Active Force Dynamics
  note: Neural Dynamics
  Motor Neuron In : Inport
  Muscle Length : Inport  Port=2
  Parameters : Inport  Port=3
  Add : Sum
  Demux : Demux  Outputs=5
  Divide : Product  Inputs=/*
  Divide1 : Product  Inputs=/*
  Divide2 : Product  Inputs=/*
  Integrator : Integrator  InitialConditionSource=external
  Integrator1 : Integrator  InitialConditionSource=external
  Subtract{,1..3} (4 alike) : Sum  Inputs=+-
  Switch : Switch  Criteria=u2 > Threshold  ZeroCross=off  SaturateOnIntegerOverflow=off  InputSameDT=off
  Zero : Constant  Value=0  OutDataTypeStr=Inherit: Inherit via back propagation
  Normalized Tension : Outport
  Activation : Outport  Port=2
  wires:
  Zero/1 -> Switch/3
  Switch/1 -> Add/2
  Divide2/1 -> Switch/1
  Muscle Length/1 -> Subtract3/1
  Parameters/1 -> Demux/1
  Motor Neuron In/1 -> Subtract/1
  Subtract/1 -> Divide/2
  Divide/1 -> Integrator/1
  Demux/3 -> Divide1/1, Divide/1
  Demux/1 -> Integrator/2
  Integrator/1 -> Subtract1/1, Subtract/2, Activation/1
  Subtract1/1 -> Divide1/2
  Divide1/1 -> Integrator1/1
  Demux/2 -> Integrator1/2
  Integrator1/1 -> Add/1, Subtract1/2
  Demux/5 -> Subtract2/1
  Demux/4 -> Subtract3/2, Subtract2/2
  Subtract2/1 -> Divide2/1
  Subtract3/1 -> Divide2/2, Switch/2
  Add/1 -> Normalized Tension/1

== system CMU_BORG_AplysiaModularNeuromechanics/Muscle Activation and Tension Module/First Order + Spring Muscle Model Template ==
  note: Neural Dynamics
  note: Active Force Dynamics
  note: Passive Force
  note: List of parameters:
      | 	- A_0: starting activation
      | 	- T_0: starting tension
      | 	- tau_i: intrinsic time constant of the muscle i
      | 	- L_0: rest length of muscle
      | 	- L_max: length of maximum force
  Motor Neuron In : Inport
  Muscle Length : Inport  Port=2
  Parameters : Inport  Port=3
  Add : Sum
  Demux : Demux  Outputs=5
  Divide : Product  Inputs=/*
  Divide1 : Product  Inputs=/*
  Divide2 : Product  Inputs=/*
  Integrator : Integrator  InitialConditionSource=external
  Integrator1 : Integrator  InitialConditionSource=external
  Subtract{,1..3} (4 alike) : Sum  Inputs=+-
  Switch : Switch  Criteria=u2 > Threshold  SaturateOnIntegerOverflow=off  InputSameDT=off
  Zero : Constant  Value=0  OutDataTypeStr=Inherit: Inherit via back propagation
  Normalized Tension : Outport
  Activation : Outport  Port=2
  wires:
  Add/1 -> Normalized Tension/1
  Subtract3/1 -> Switch/2, Divide2/2
  Subtract2/1 -> Divide2/1
  Demux/4 -> Subtract2/2, Subtract3/2
  Demux/5 -> Subtract2/1
  Integrator1/1 -> Subtract1/2, Add/1
  Demux/2 -> Integrator1/2
  Divide1/1 -> Integrator1/1
  Subtract1/1 -> Divide1/2
  Integrator/1 -> Activation/1, Subtract/2, Subtract1/1
  Demux/1 -> Integrator/2
  Demux/3 -> Divide/1, Divide1/1
  Divide/1 -> Integrator/1
  Subtract/1 -> Divide/2
  Motor Neuron In/1 -> Subtract/1
  Parameters/1 -> Demux/1
  Muscle Length/1 -> Subtract3/1
  Divide2/1 -> Switch/1
  Switch/1 -> Add/2
  Zero/1 -> Switch/3

== system CMU_BORG_AplysiaModularNeuromechanics/Muscle Activation and Tension Module/First Order Muscle Model Template ==
  note: Neural Dynamics
  note: List of parameters:
      | 	- A_0: starting activation
      | 	- T_0: starting tension
      | 	- tau_i: intrinsic time constant of the muscle i
  note: Force Dynamics
  Motor Neuron In : Inport
  Muscle Length : Inport  Port=2
  Parameters : Inport  Port=3
  Demux : Demux  Outputs=3
  Divide : Product  Inputs=/*
  Divide1 : Product  Inputs=/*
  Integrator : Integrator  InitialConditionSource=external
  Integrator1 : Integrator  InitialConditionSource=external
  Subtract : Sum  Inputs=+-
  Subtract1 : Sum  Inputs=+-
  Terminator : Terminator
  Normalized Tension : Outport
  Activation : Outport  Port=2
  wires:
  Muscle Length/1 -> Terminator/1
  Parameters/1 -> Demux/1
  Motor Neuron In/1 -> Subtract/1
  Subtract/1 -> Divide/2
  Divide/1 -> Integrator/1
  Demux/3 -> Divide1/1, Divide/1
  Demux/1 -> Integrator/2
  Integrator/1 -> Subtract1/1, Subtract/2, Activation/1
  Subtract1/1 -> Divide1/2
  Divide1/1 -> Integrator1/1
  Demux/2 -> Integrator1/2
  Integrator1/1 -> Subtract1/2, Normalized Tension/1

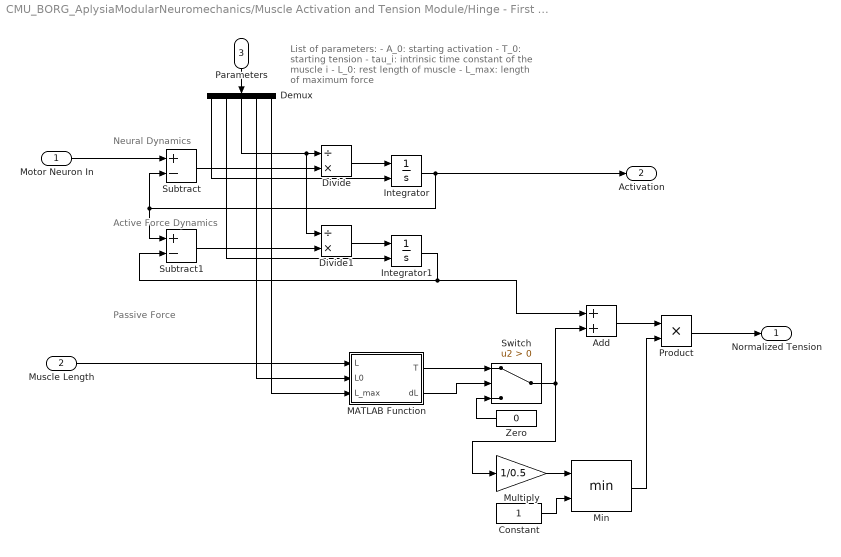
== system CMU_BORG_AplysiaModularNeuromechanics/Muscle Activation and Tension Module/Hinge - First Order + Spring Muscle Model ==
  note: Neural Dynamics
  note: Active Force Dynamics
  note: Passive Force
  note: List of parameters:
      | 	- A_0: starting activation
      | 	- T_0: starting tension
      | 	- tau_i: intrinsic time constant of the muscle i
      | 	- L_0: rest length of muscle
      | 	- L_max: length of maximum force
  Motor Neuron In : Inport
  Muscle Length : Inport  Port=2
  Parameters : Inport  Port=3
  Add : Sum
  Constant : Constant
  Demux : Demux  Outputs=5
  Divide : Product  Inputs=/*
  Divide1 : Product  Inputs=/*
  Integrator : Integrator  InitialConditionSource=external
  Integrator1 : Integrator  InitialConditionSource=external
  MATLAB Function : MATLAB Function  TreatAsAtomicUnit=on
  Min : MinMax  Inputs=2
  Multiply : Gain  Gain=1/0.5
  Product : Product
  Subtract : Sum  Inputs=+-
  Subtract1 : Sum  Inputs=+-
  Switch : Switch  Criteria=u2 > Threshold  ZeroCross=off  SaturateOnIntegerOverflow=off  InputSameDT=off
  Zero : Constant  Value=0  OutDataTypeStr=Inherit: Inherit via back propagation
  Normalized Tension : Outport
  Activation : Outport  Port=2
  wires:
  Demux/4 -> MATLAB Function/2(L0)
  Demux/5 -> MATLAB Function/3(L_max)
  Integrator1/1 -> Subtract1/2, Add/1
  Demux/2 -> Integrator1/2
  Divide1/1 -> Integrator1/1
  Subtract1/1 -> Divide1/2
  Integrator/1 -> Activation/1, Subtract/2, Subtract1/1
  Demux/1 -> Integrator/2
  Demux/3 -> Divide/1, Divide1/1
  Divide/1 -> Integrator/1
  Subtract/1 -> Divide/2
  Motor Neuron In/1 -> Subtract/1
  Parameters/1 -> Demux/1
  Muscle Length/1 -> MATLAB Function/1(L)
  Zero/1 -> Switch/3
  MATLAB Function/1(T) -> Switch/1
  MATLAB Function/2(dL) -> Switch/2
  Switch/1 -> Add/2, Multiply/1
  Add/1 -> Product/1
  Product/1 -> Normalized Tension/1
  Constant/1 -> Min/2
  Min/1 -> Product/2
  Multiply/1 -> Min/1

== system CMU_BORG_AplysiaModularNeuromechanics/Muscle Activation and Tension Module/I1d - First Order + Spring Muscle Model ==
  note: Neural Dynamics
  note: Active Force Dynamics
  note: Passive Force
  note: List of parameters:
      | 	- A_0: starting activation
      | 	- T_0: starting tension
      | 	- tau_i: intrinsic time constant of the muscle i
      | 	- L_0: rest length of muscle
      | 	- L_max: length of maximum force
  Motor Neuron In : Inport
  Muscle Length : Inport  Port=2
  Parameters : Inport  Port=3
  Add : Sum
  Demux : Demux  Outputs=5
  Divide : Product  Inputs=/*
  Divide1 : Product  Inputs=/*
  Divide2 : Product  Inputs=/*
  Integrator : Integrator  InitialConditionSource=external
  Integrator1 : Integrator  InitialConditionSource=external
  Subtract{,1..3} (4 alike) : Sum  Inputs=+-
  Normalized Tension : Outport
  Activation : Outport  Port=2
  wires:
  Add/1 -> Normalized Tension/1
  Subtract3/1 -> Divide2/2
  Subtract2/1 -> Divide2/1
  Demux/4 -> Subtract2/2, Subtract3/2
  Demux/5 -> Subtract2/1
  Integrator1/1 -> Add/1, Subtract1/2
  Demux/2 -> Integrator1/2
  Divide1/1 -> Integrator1/1
  Subtract1/1 -> Divide1/2
  Integrator/1 -> Activation/1, Subtract/2, Subtract1/1
  Demux/1 -> Integrator/2
  Demux/3 -> Divide/1, Divide1/1
  Divide/1 -> Integrator/1
  Subtract/1 -> Divide/2
  Motor Neuron In/1 -> Subtract/1
  Parameters/1 -> Demux/1
  Muscle Length/1 -> Subtract3/1
  Divide2/1 -> Add/2

== system CMU_BORG_AplysiaModularNeuromechanics/Muscle Activation and Tension Module/I1v - First Order + Spring Muscle Model ==
  note: List of parameters:
      | 	- A_0: starting activation
      | 	- T_0: starting tension
      | 	- tau_i: intrinsic time constant of the muscle i
      | 	- L_0: rest length of muscle
      | 	- L_max: length of maximum force
  note: Passive Force
  note: Active Force Dynamics
  note: Neural Dynamics
  Motor Neuron In : Inport
  Muscle Length : Inport  Port=2
  Parameters : Inport  Port=3
  Add : Sum
  Demux : Demux  Outputs=5
  Divide : Product  Inputs=/*
  Divide1 : Product  Inputs=/*
  Divide2 : Product  Inputs=/*
  Integrator : Integrator  InitialConditionSource=external
  Integrator1 : Integrator  InitialConditionSource=external
  Subtract{,1..3} (4 alike) : Sum  Inputs=+-
  Normalized Tension : Outport
  Activation : Outport  Port=2
  wires:
  Divide2/1 -> Add/2
  Parameters/1 -> Demux/1
  Motor Neuron In/1 -> Subtract/1
  Subtract/1 -> Divide/2
  Divide/1 -> Integrator/1
  Demux/3 -> Divide1/1, Divide/1
  Demux/1 -> Integrator/2
  Integrator/1 -> Subtract1/1, Subtract/2, Activation/1
  Subtract1/1 -> Divide1/2
  Divide1/1 -> Integrator1/1
  Demux/2 -> Integrator1/2
  Demux/5 -> Subtract2/1
  Subtract2/1 -> Divide2/1
  Subtract3/1 -> Divide2/2
  Add/1 -> Normalized Tension/1
  Integrator1/1 -> Add/1, Subtract1/2
  Muscle Length/1 -> Subtract3/1
  Demux/4 -> Subtract3/2, Subtract2/2

== system CMU_BORG_AplysiaModularNeuromechanics/Muscle Activation and Tension Module/I2 - First Order + Spring Muscle Model2 ==
  note: List of parameters:
      | 	- A_0: starting activation
      | 	- T_0: starting tension
      | 	- tau_i: intrinsic time constant of the muscle i
      | 	- L_0: rest length of muscle
      | 	- L_max: length of maximum force
  note: Passive Force
  note: Active Force Dynamics
  note: Neural Dynamics
  Motor Neuron In : Inport
  Muscle Length : Inport  Port=2
  Parameters : Inport  Port=3
  Add : Sum
  Demux : Demux  Outputs=5
  Divide : Product  Inputs=/*
  Divide1 : Product  Inputs=/*
  Divide2 : Product  Inputs=/*
  Integrator : Integrator  InitialConditionSource=external
  Integrator1 : Integrator  InitialConditionSource=external
  Subtract{,1..3} (4 alike) : Sum  Inputs=+-
  Switch : Switch  Criteria=u2 > Threshold  ZeroCross=off  SaturateOnIntegerOverflow=off  InputSameDT=off
  Zero : Constant  Value=0  OutDataTypeStr=Inherit: Inherit via back propagation
  Normalized Tension : Outport
  Activation : Outport  Port=2
  wires:
  Zero/1 -> Switch/3
  Switch/1 -> Add/2
  Divide2/1 -> Switch/1
  Muscle Length/1 -> Subtract3/1
  Parameters/1 -> Demux/1
  Motor Neuron In/1 -> Subtract/1
  Subtract/1 -> Divide/2
  Divide/1 -> Integrator/1
  Demux/3 -> Divide1/1, Divide/1
  Demux/1 -> Integrator/2
  Integrator/1 -> Subtract1/1, Subtract/2, Activation/1
  Subtract1/1 -> Divide1/2
  Divide1/1 -> Integrator1/1
  Demux/2 -> Integrator1/2
  Integrator1/1 -> Add/1, Subtract1/2
  Demux/5 -> Subtract2/1
  Demux/4 -> Subtract3/2, Subtract2/2
  Subtract2/1 -> Divide2/1
  Subtract3/1 -> Divide2/2, Switch/2
  Add/1 -> Normalized Tension/1

== system CMU_BORG_AplysiaModularNeuromechanics/Muscle Activation and Tension Module/I2 Param Updates1 ==
  In params : Inport
  CBI3 : Inport  Port=2
  Demux : Demux  Outputs=6
  Mux : Mux  Inputs=5
  Switch : Switch  Criteria=u2 > Threshold  Threshold=0.5  SaturateOnIntegerOverflow=off  InputSameDT=off
  Out params : Outport
  wires:
  In params/1 -> Demux/1
  Mux/1 -> Out params/1
  Demux/1 -> Mux/1
  Demux/2 -> Mux/2
  Demux/5 -> Mux/4
  Demux/6 -> Mux/5
  Demux/3 -> Switch/1  "tau_ingestive"
  Demux/4 -> Switch/3  "tau_egestive"
  CBI3/1 -> Switch/2
  Switch/1 -> Mux/3

== system CMU_BORG_AplysiaModularNeuromechanics/Muscle Activation and Tension Module/I3 (anterior) - First Order Muscle Model ==
  note: Force Dynamics
  note: List of parameters:
      | 	- A_0: starting activation
      | 	- T_0: starting tension
      | 	- tau_i: intrinsic time constant of the muscle i
  note: Neural Dynamics
  Motor Neuron In : Inport
  Muscle Length : Inport  Port=2
  Parameters : Inport  Port=3
  Demux : Demux  Outputs=3
  Divide : Product  Inputs=/*
  Divide1 : Product  Inputs=/*
  Integrator : Integrator  InitialConditionSource=external
  Integrator1 : Integrator  InitialConditionSource=external
  Subtract : Sum  Inputs=+-
  Subtract1 : Sum  Inputs=+-
  Terminator : Terminator
  Normalized Tension : Outport
  Activation : Outport  Port=2
  wires:
  Integrator1/1 -> Normalized Tension/1, Subtract1/2
  Demux/2 -> Integrator1/2
  Divide1/1 -> Integrator1/1
  Subtract1/1 -> Divide1/2
  Integrator/1 -> Activation/1, Subtract/2, Subtract1/1
  Demux/1 -> Integrator/2
  Demux/3 -> Divide/1, Divide1/1
  Divide/1 -> Integrator/1
  Subtract/1 -> Divide/2
  Motor Neuron In/1 -> Subtract/1
  Parameters/1 -> Demux/1
  Muscle Length/1 -> Terminator/1

== system CMU_BORG_AplysiaModularNeuromechanics/Muscle Activation and Tension Module/I3 - First Order Muscle Model ==
  note: Neural Dynamics
  note: List of parameters:
      | 	- A_0: starting activation
      | 	- T_0: starting tension
      | 	- tau_i: intrinsic time constant of the muscle i
  note: Force Dynamics
  Motor Neuron In : Inport
  Muscle Length : Inport  Port=2
  Parameters : Inport  Port=3
  Demux : Demux  Outputs=3
  Divide : Product  Inputs=/*
  Divide1 : Product  Inputs=/*
  Integrator : Integrator  InitialConditionSource=external
  Integrator1 : Integrator  InitialConditionSource=external
  Subtract : Sum  Inputs=+-
  Subtract1 : Sum  Inputs=+-
  Terminator : Terminator
  Normalized Tension : Outport
  Activation : Outport  Port=2
  wires:
  Muscle Length/1 -> Terminator/1
  Parameters/1 -> Demux/1
  Motor Neuron In/1 -> Subtract/1
  Subtract/1 -> Divide/2
  Divide/1 -> Integrator/1
  Demux/3 -> Divide1/1, Divide/1
  Demux/1 -> Integrator/2
  Integrator/1 -> Subtract1/1, Subtract/2, Activation/1
  Subtract1/1 -> Divide1/2
  Divide1/1 -> Integrator1/1
  Demux/2 -> Integrator1/2
  Integrator1/1 -> Subtract1/2, Normalized Tension/1

== system CMU_BORG_AplysiaModularNeuromechanics/Muscle Activation and Tension Module/I4 - First Order Muscle Model ==
  note: Force Dynamics
  note: List of parameters:
      | 	- A_0: starting activation
      | 	- T_0: starting tension
      | 	- tau_i: intrinsic time constant of the muscle i
  note: Neural Dynamics
  Motor Neuron In : Inport
  Muscle Length : Inport  Port=2
  Parameters : Inport  Port=3
  Demux : Demux  Outputs=3
  Divide : Product  Inputs=/*
  Divide1 : Product  Inputs=/*
  Integrator : Integrator  InitialConditionSource=external
  Integrator1 : Integrator  InitialConditionSource=external
  Subtract : Sum  Inputs=+-
  Subtract1 : Sum  Inputs=+-
  Terminator : Terminator
  Normalized Tension : Outport
  Activation : Outport  Port=2
  wires:
  Integrator1/1 -> Normalized Tension/1, Subtract1/2
  Demux/2 -> Integrator1/2
  Divide1/1 -> Integrator1/1
  Subtract1/1 -> Divide1/2
  Integrator/1 -> Activation/1, Subtract/2, Subtract1/1
  Demux/1 -> Integrator/2
  Demux/3 -> Divide/1, Divide1/1
  Divide/1 -> Integrator/1
  Subtract/1 -> Divide/2
  Motor Neuron In/1 -> Subtract/1
  Parameters/1 -> Demux/1
  Muscle Length/1 -> Terminator/1

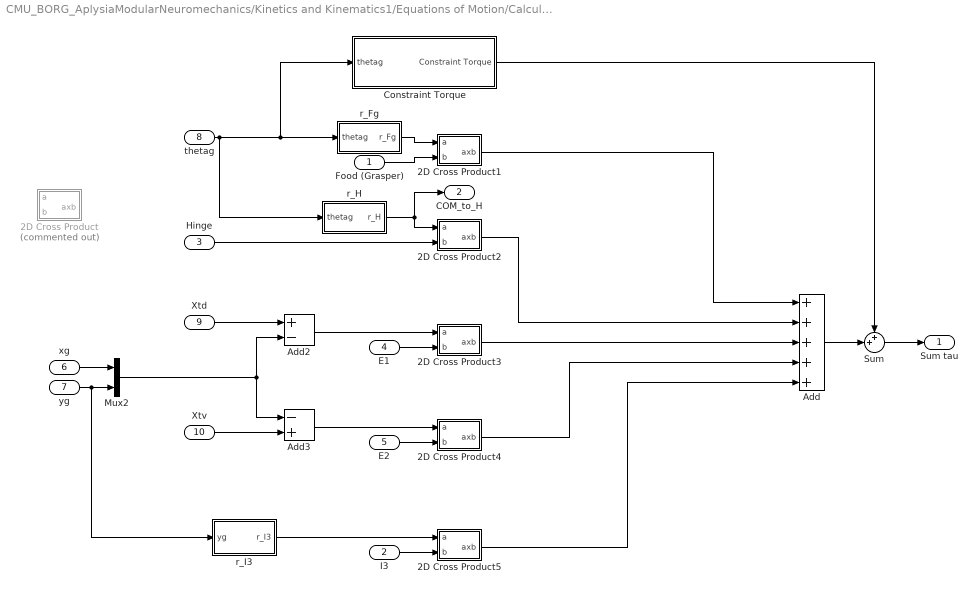
== system CMU_BORG_AplysiaModularNeuromechanics/Kinetics and Kinematics1/Equations of Motion/Calculate Sum of Torques ==
  Food (Grasper) : Inport
  I3 : Inport  Port=2
  Hinge : Inport  Port=3
  E1 : Inport  Port=4
  E2 : Inport  Port=5
  xg : Inport  Port=6
  yg : Inport  Port=7
  thetag : Inport  Port=8
  Xtd : Inport  Port=9
  Xtv : Inport  Port=10
  2D Cross Product : Subsystem  Commented=on
  2D Cross Product1 : Subsystem
  2D Cross Product2 : Subsystem
  2D Cross Product3 : Subsystem
  2D Cross Product4 : Subsystem
  2D Cross Product5 : Subsystem
  Add : Sum  Inputs=+++++
  Add2 : Sum  Inputs=+-
  Add3 : Sum  Inputs=-+
  Constraint Torque : Subsystem
  Mux2 : Mux  Inputs=2
  Sum : Sum  Inputs=++|
  r_Fg : Subsystem
  r_H : Subsystem
  r_I3 : Subsystem
  Sum tau : Outport
  COM_to_H : Outport  Port=2
  wires:
  Food (Grasper)/1 -> 2D Cross Product1/2(b)
  thetag/1 -> Constraint Torque/1(thetag), r_Fg/1(thetag), r_H/1(thetag)
  r_H/1(r_H) -> 2D Cross Product2/1(a), COM_to_H/1
  E1/1 -> 2D Cross Product3/2(b)
  xg/1 -> Mux2/1
  yg/1 -> r_I3/1(yg), Mux2/2
  Mux2/1 -> Add3/1, Add2/2
  Add2/1 -> 2D Cross Product3/1(a)
  E2/1 -> 2D Cross Product4/2(b)
  Add3/1 -> 2D Cross Product4/1(a)
  I3/1 -> 2D Cross Product5/2(b)
  r_I3/1(r_I3) -> 2D Cross Product5/1(a)
  2D Cross Product3/1(axb) -> Add/3
  2D Cross Product1/1(axb) -> Add/1
  2D Cross Product2/1(axb) -> Add/2
  2D Cross Product4/1(axb) -> Add/4
  2D Cross Product5/1(axb) -> Add/5
  Xtd/1 -> Add2/1
  Xtv/1 -> Add3/2
  r_Fg/1(r_Fg) -> 2D Cross Product1/1(a)
  Add/1 -> Sum/2
  Sum/1 -> Sum tau/1
  Constraint Torque/1(Constraint Torque) -> Sum/1
  Hinge/1 -> 2D Cross Product2/2(b)

== system CMU_BORG_AplysiaModularNeuromechanics/Kinetics and Kinematics1/Equations of Motion/Solving for Lagrange Multiplier ==
  yg : Inport
  R_hat : Inport  Port=2
  theta_h : Inport  Port=3
  theta_g : Inport  Port=4
  Constant2 : Constant  Value=C_theta
  Constraint Derivatives : MATLAB Function  TreatAsAtomicUnit=on
  Divide : Product  Inputs=*/
  Gain : Gain  Gain=C_yg
  Square : Math  Operator=square
  Sum : Sum  Inputs=++|
  del_factor : Outport
  denom : Outport  Port=2
  wires:
  Constraint Derivatives/1(dfdtheta) -> Divide/1
  Constraint Derivatives/2(dfdy) -> Divide/2
  Divide/1 -> Square/1, del_factor/1
  yg/1 -> Constraint Derivatives/1(yg)
  theta_g/1 -> Constraint Derivatives/2(theta_g)
  R_hat/1 -> Constraint Derivatives/3(R)
  theta_h/1 -> Constraint Derivatives/4(theta_H)
  Constant2/1 -> Sum/2
  Gain/1 -> Sum/1
  Square/1 -> Gain/1
  Sum/1 -> denom/1
